simulink model "pointcloud2_test"  (R2021b)
settings: Solver=FixedStepAuto  StartTime=0.0  StopTime=10.0  RelTol=1e-3
model workspace (MAT data in the model file):
  Logfile_Data_Object = ros2bag
  Logfile_Data_Object.FilePath = 'C:\azumiken\lidars_point_raw\lidars_point_raw_0.db3'
  Logfile_Data_Object.StartTime = 1633675920681641206
  Logfile_Data_Object.EndTime = 1633676017682751873
  Logfile_Data_Object.AvailableTopics = table
  Logfile_Data_Object.AvailableTopics.data{1} = [969; 970]
  Logfile_Data_Object.AvailableTopics.data{2} = categorical
  Logfile_Data_Object.AvailableTopics.data{2}.categoryNames = {'sensor_msgs/PointCloud2'}
  Logfile_Data_Object.AvailableTopics.data{2}.codes = [1; 1]
  Logfile_Data_Object.AvailableTopics.data{3}{1} = '% contain additional information such as normals, intensity, etc. The
    | % point data is stored as a binary blob, its layout described by the
    | % contents of the "fields" array.
    | %
    | % The point cloud data may be organized 2d (image-like) or 1d (unordered).
    | % Point clouds organized as 2d images may be produced by camera depth sensors
    | % such as stereo or Time-of-flight.
    | 
    | % Time of sensor data acquisition, and the coordinate frame ID (for 3d points).
    | std_msgs/Header header
    | 
    | % 2D structure of the point cloud. If the cloud is unordered, height is
    | % 1 and width is the length of the point cloud.
    | uint32 height
    | uint32 width
    | 
    | % Describes the channels and their layout in the binary data blob.
    | PointField[] fields
    | 
    | logical    is_bigendian % Is this data bigendian?
    | uint32  point_step      % Length of a point in bytes
    | uint32  row_step        % Length of a row in bytes
    | uint8[] data            % Actual point data, size is (row_step*height)
    | 
    | logical is_dense        % True if there are no invalid points'
  Logfile_Data_Object.AvailableTopics.data{3}{2} = '% contain additional information such as normals, intensity, etc. The
    | % point data is stored as a binary blob, its layout described by the
    | % contents of the "fields" array.
    | %
    | % The point cloud data may be organized 2d (image-like) or 1d (unordered).
    | % Point clouds organized as 2d images may be produced by camera depth sensors
    | % such as stereo or Time-of-flight.
    | 
    | % Time of sensor data acquisition, and the coordinate frame ID (for 3d points).
    | std_msgs/Header header
    | 
    | % 2D structure of the point cloud. If the cloud is unordered, height is
    | % 1 and width is the length of the point cloud.
    | uint32 height
    | uint32 width
    | 
    | % Describes the channels and their layout in the binary data blob.
    | PointField[] fields
    | 
    | logical    is_bigendian % Is this data bigendian?
    | uint32  point_step      % Length of a point in bytes
    | uint32  row_step        % Length of a row in bytes
    | uint8[] data            % Actual point data, size is (row_step*height)
    | 
    | logical is_dense        % True if there are no invalid points'
  Logfile_Data_Object.AvailableTopics.ndims = 2
  Logfile_Data_Object.AvailableTopics.nrows = 2
  Logfile_Data_Object.AvailableTopics.rownames = {'/lidar_front/points_raw'; '/lidar_rear/points_raw'}
  Logfile_Data_Object.AvailableTopics.nvars = 3
  Logfile_Data_Object.AvailableTopics.varnames = {'NumMessages', 'MessageType', 'MessageDefinition'}
  Logfile_Data_Object.AvailableTopics.props.useVariableNamesOriginal = 0
  Logfile_Data_Object.AvailableTopics.props.useDimensionNamesOriginal = 0
  Logfile_Data_Object.AvailableTopics.props.CustomProps = struct()
  Logfile_Data_Object.AvailableTopics.props.VariableCustomProps = struct()
  Logfile_Data_Object.AvailableTopics.props.versionSavedFrom = 4
  Logfile_Data_Object.AvailableTopics.props.minCompatibleVersion = 1
  Logfile_Data_Object.AvailableTopics.props.incompatibilityMsg = ''
  Logfile_Data_Object.AvailableTopics.props.VersionSavedFrom = 4
  Logfile_Data_Object.AvailableTopics.props.Description = ''
  Logfile_Data_Object.AvailableTopics.props.VariableNamesOriginal = {}
  Logfile_Data_Object.AvailableTopics.props.DimensionNames = {'Row', 'Variables'}
  Logfile_Data_Object.AvailableTopics.props.DimensionNamesOriginal = {}
  Logfile_Data_Object.AvailableTopics.props.UserData = []
  Logfile_Data_Object.AvailableTopics.props.VariableDescriptions = {}
  Logfile_Data_Object.AvailableTopics.props.VariableUnits = {}
  Logfile_Data_Object.AvailableTopics.props.VariableContinuity = {}
  Logfile_Data_Object.MessageList = table
  Logfile_Data_Object.MessageList.data{1} = [1633675920681641206 1633675920704850047 1633675920710280571 1633675920841302537 1633675920849007917 1633675920944718285 1633675920950454411 1633675921046456357 1633675921051238695 1633675921143527086 1633675921154682295 1633675921262758351 ... (1939 elements, 1939x1)]
  Logfile_Data_Object.MessageList.data{2} = categorical
  Logfile_Data_Object.MessageList.data{2}.categoryNames = {'/lidar_rear/points_raw'; '/lidar_front/points_raw'}
  Logfile_Data_Object.MessageList.data{2}.codes = [1 2 1 2 1 2 1 2 1 2 1 2 ... (1939 elements, 1939x1)]
  Logfile_Data_Object.MessageList.data{3} = categorical
  Logfile_Data_Object.MessageList.data{3}.categoryNames = {'sensor_msgs/PointCloud2'}
  Logfile_Data_Object.MessageList.data{3}.codes = [1 1 1 1 1 1 1 1 1 1 1 1 ... (1939 elements, 1939x1)]
  Logfile_Data_Object.MessageList.ndims = 2
  Logfile_Data_Object.MessageList.nrows = 1939
  Logfile_Data_Object.MessageList.nvars = 3
  Logfile_Data_Object.MessageList.varnames = {'Time', 'Topic', 'MessageType'}
  Logfile_Data_Object.MessageList.props.useVariableNamesOriginal = 0
  Logfile_Data_Object.MessageList.props.useDimensionNamesOriginal = 0
  Logfile_Data_Object.MessageList.props.CustomProps = struct()
  Logfile_Data_Object.MessageList.props.VariableCustomProps = struct()
  Logfile_Data_Object.MessageList.props.versionSavedFrom = 4
  Logfile_Data_Object.MessageList.props.minCompatibleVersion = 1
  Logfile_Data_Object.MessageList.props.incompatibilityMsg = ''
  Logfile_Data_Object.MessageList.props.VersionSavedFrom = 4
  Logfile_Data_Object.MessageList.props.Description = ''
  Logfile_Data_Object.MessageList.props.VariableNamesOriginal = {}
  Logfile_Data_Object.MessageList.props.DimensionNames = {'Row', 'Variables'}
  Logfile_Data_Object.MessageList.props.DimensionNamesOriginal = {}
  Logfile_Data_Object.MessageList.props.UserData = []
  Logfile_Data_Object.MessageList.props.VariableDescriptions = {}
  Logfile_Data_Object.MessageList.props.VariableUnits = {}
  Logfile_Data_Object.MessageList.props.VariableContinuity = {}
  Logfile_Data_Object.TopicTypeMap = containers.Map
  Logfile_Data_Object.TopicTypeMap.serialization.keys = {'/lidar_front/points_raw', '/lidar_rear/points_raw'}
  Logfile_Data_Object.TopicTypeMap.serialization.values = {'sensor_msgs/PointCloud2', 'sensor_msgs/PointCloud2'}
  Logfile_Data_Object.TopicTypeMap.serialization.uniformity = 1
  Logfile_Data_Object.TopicTypeMap.serialization.keyType = 'char'
  Logfile_Data_Object.TopicTypeMap.serialization.valueType = 'char'
  Logfile_Data_Object.TopicDefinitionMap = containers.Map
  Logfile_Data_Object.TopicDefinitionMap.serialization.keys = {'/lidar_front/points_raw', '/lidar_rear/points_raw'}
  Logfile_Data_Object.TopicDefinitionMap.serialization.values{1} = '% contain additional information such as normals, intensity, etc. The
    | % point data is stored as a binary blob, its layout described by the
    | % contents of the "fields" array.
    | %
    | % The point cloud data may be organized 2d (image-like) or 1d (unordered).
    | % Point clouds organized as 2d images may be produced by camera depth sensors
    | % such as stereo or Time-of-flight.
    | 
    | % Time of sensor data acquisition, and the coordinate frame ID (for 3d points).
    | std_msgs/Header header
    | 
    | % 2D structure of the point cloud. If the cloud is unordered, height is
    | % 1 and width is the length of the point cloud.
    | uint32 height
    | uint32 width
    | 
    | % Describes the channels and their layout in the binary data blob.
    | PointField[] fields
    | 
    | logical    is_bigendian % Is this data bigendian?
    | uint32  point_step      % Length of a point in bytes
    | uint32  row_step        % Length of a row in bytes
    | uint8[] data            % Actual point data, size is (row_step*height)
    | 
    | logical is_dense        % True if there are no invalid points'
  Logfile_Data_Object.TopicDefinitionMap.serialization.values{2} = '% contain additional information such as normals, intensity, etc. The
    | % point data is stored as a binary blob, its layout described by the
    | % contents of the "fields" array.
    | %
    | % The point cloud data may be organized 2d (image-like) or 1d (unordered).
    | % Point clouds organized as 2d images may be produced by camera depth sensors
    | % such as stereo or Time-of-flight.
    | 
    | % Time of sensor data acquisition, and the coordinate frame ID (for 3d points).
    | std_msgs/Header header
    | 
    | % 2D structure of the point cloud. If the cloud is unordered, height is
    | % 1 and width is the length of the point cloud.
    | uint32 height
    | uint32 width
    | 
    | % Describes the channels and their layout in the binary data blob.
    | PointField[] fields
    | 
    | logical    is_bigendian % Is this data bigendian?
    | uint32  point_step      % Length of a point in bytes
    | uint32  row_step        % Length of a row in bytes
    | uint8[] data            % Actual point data, size is (row_step*height)
    | 
    | logical is_dense        % True if there are no invalid points'
  Logfile_Data_Object.TopicDefinitionMap.serialization.uniformity = 1
  Logfile_Data_Object.TopicDefinitionMap.serialization.keyType = 'char'
  Logfile_Data_Object.TopicDefinitionMap.serialization.valueType = 'char'
  Logfile_Path = 'C:\azumiken\lidars_point_raw\lidars_point_raw_0.db3'
  Logfile_Playback_Duration = nan
  Logfile_Playback_Offset = nan
  SL_ROS_VariableLengthArrays_MaxSizes.CommonInfo.ArrayTruncateAction = 'EmitWarning'
  SL_ROS_VariableLengthArrays_MaxSizes.MsgTypeMap = containers.Map
  SL_ROS_VariableLengthArrays_MaxSizes.MsgTypeMap.serialization.keys = {'sensor_msgs/PointCloud2'}
  SL_ROS_VariableLengthArrays_MaxSizes.MsgTypeMap.serialization.values{1}(1).PropertyName = 'data'
  SL_ROS_VariableLengthArrays_MaxSizes.MsgTypeMap.serialization.values{1}(1).DataType = 'uint8'
  SL_ROS_VariableLengthArrays_MaxSizes.MsgTypeMap.serialization.values{1}(1).MaxLength = 55000
  SL_ROS_VariableLengthArrays_MaxSizes.MsgTypeMap.serialization.values{1}(2).PropertyName = 'fields'
  SL_ROS_VariableLengthArrays_MaxSizes.MsgTypeMap.serialization.values{1}(2).DataType = 'sensor_msgs/PointField'
  SL_ROS_VariableLengthArrays_MaxSizes.MsgTypeMap.serialization.values{1}(2).MaxLength = 16
  SL_ROS_VariableLengthArrays_MaxSizes.MsgTypeMap.serialization.uniformity = 0
  SL_ROS_VariableLengthArrays_MaxSizes.MsgTypeMap.serialization.keyType = 'char'
  SL_ROS_VariableLengthArrays_MaxSizes.MsgTypeMap.serialization.valueType = 'any'
libraries: ros2lib x2
settings Model: Creator=takum  LastModifiedBy=takum
settings OptimizationCC: EnhancedBackFolding=on  PassReuseOutputArgsAs=Individual arguments  ZeroExternalMemoryAtStartup=off  ZeroInternalMemoryAtStartup=off  MaxStackSize=64  OptimizeBlockOrder=speed  DifferentSizesBufferReuse=on  OptimizationCustomize=off  EfficientTunableParamExpr=on
settings DebuggingCC: ParameterTunabilityLossMsg=error  UnderSpecifiedDimensionMsg=error
settings SFSimCC: MATLABDynamicMemAlloc=off
settings RTWCC: Description=Embedded Coder  SystemTargetFile=ert.tlc  HardwareBoard=Robot Operating System 2 (ROS 2)  TemplateMakefile=ert_default_tmf  Toolchain=Colcon Tools  TargetLang=C++
settings CodeAppCC: ForceParamTrailComments=on  IgnoreCustomStorageClasses=off  OperatorAnnotations=on  SimulinkDataObjDesc=on  SFDataObjDesc=on  InsertBlockDesc=on
settings ERTTargetCC: CodeInterfacePackaging=C++ class  RootIOFormat=Structure reference

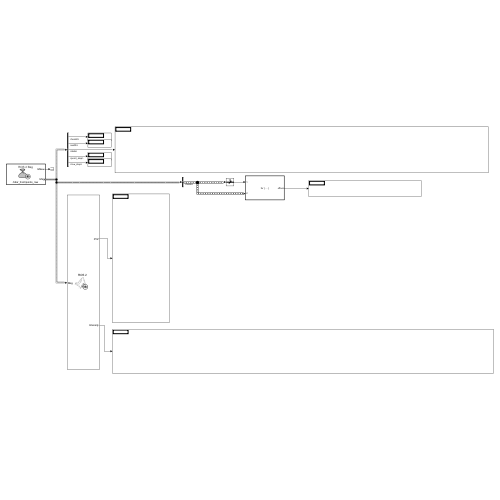
[thumbnail: Simulink's stored preview of the top-level diagram]
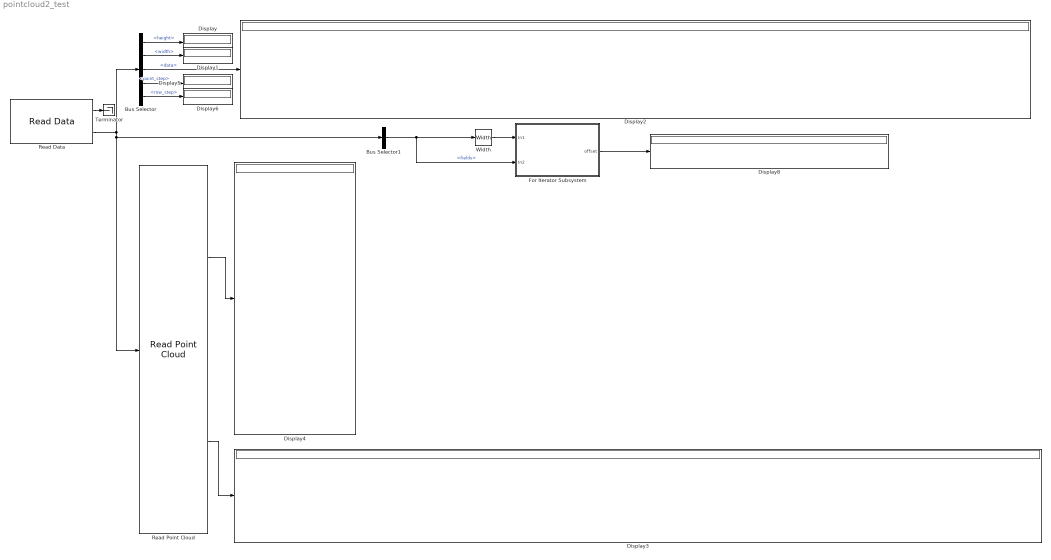
== system pointcloud2_test ==
  Bus Selector : BusSelector  OutputSignals=height,width,data,point_step,row_step
  Bus Selector1 : BusSelector  OutputSignals=fields
  Display{,1..6,8} (8 alike) : Display
  For Iterator Subsystem : Subsystem  TreatAsAtomicUnit=on
  Read Data : ros2lib/Read Data  topic=/lidar_front/points_raw  sampleTime=-1  logfileType=rosbag2  modelName=pointcloud2_test  msgType=sensor_msgs/PointCloud2
      settings: SourceProductBaseCode=RR
  Read Point Cloud : ros2lib/Read Point Cloud  MaximumPointCloudSize=[1, 55000]  PreserveStructure=off  ShowRGBOutput=off  ShowIntensityOutput=on  ShowErrorCodeOutput=off  VariableSizeOutputs=off
      settings: SourceProductBaseCode=RR
  Terminator : Terminator
  Width : Width
  wires:
  Read Data/2 -> Bus Selector1/1, Read Point Cloud/1, Bus Selector/1
  Read Data/1 -> Terminator/1
  Bus Selector/1 -> Display/1  "<height>"
  Bus Selector/2 -> Display1/1  "<width>"
  Bus Selector/3 -> Display2/1  "<data>"
  Read Point Cloud/2 -> Display3/1
  Read Point Cloud/1 -> Display4/1
  Bus Selector/4 -> Display5/1  "<point_step>"
  Bus Selector/5 -> Display6/1  "<row_step>"
  Bus Selector1/1 -> For Iterator Subsystem/2(In2), Width/1  "<fields>"
  Width/1 -> For Iterator Subsystem/1(In1)
  For Iterator Subsystem/1(offset) -> Display8/1

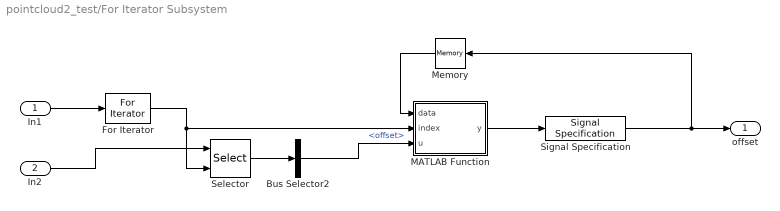
== system pointcloud2_test/For Iterator Subsystem ==
  In1 : Inport
  In2 : Inport  Port=2
  Bus Selector2 : BusSelector  OutputSignals=offset
  For Iterator : ForIterator  IterationSource=external
  MATLAB Function : MATLAB Function  TreatAsAtomicUnit=on
  Memory : Memory  InheritSampleTime=on
  Selector : Selector  InputPortWidth=16  IndexOptions=Starting index (port)  Indices=[1 3]  OutputSizes=1
  Signal Specification : SignalSpecification  Dimensions=1*16
  offset : Outport
  wires:
  In1/1 -> For Iterator/1
  Selector/1 -> Bus Selector2/1
  In2/1 -> Selector/1
  Bus Selector2/1 -> MATLAB Function/3(u)  "<offset>"
  MATLAB Function/1(y) -> Signal Specification/1
  Memory/1 -> MATLAB Function/1(data)
  Signal Specification/1 -> Memory/1, offset/1
  For Iterator/1 -> MATLAB Function/2(index), Selector/2

== matlab function pointcloud2_test/For Iterator Subsystem/MATLAB Function ==
  data: data input; index input; u input; y output
function y = fcn(data, index, u)
data(index)=u
y=data;
